simulink model "Practica5"  (R2020b)
settings: Solver=VariableStepAuto  StartTime=0.0  StopTime=10.0  RelTol=1e-3
values from neighbouring files (symbols this model uses):
  Cf = 0.0024    [Practica5Script.m]
  Fr = [10;0]    [Practica5Script.m]
  I = 0.0016    [Practica5Script.m]
  Ka = Ka(1)    [Practica5Script.m]
  Kd = [500 0;0 500]    [Practica5Script.m]
  Kp = Kp(1)    [Practica5Script.m]
  P = 0.00064    [Practica5Script.m]
undefined symbols (not defined in the file or in its folder): K, xe
settings Model: Creator=Danie  LastModifiedBy=Danie

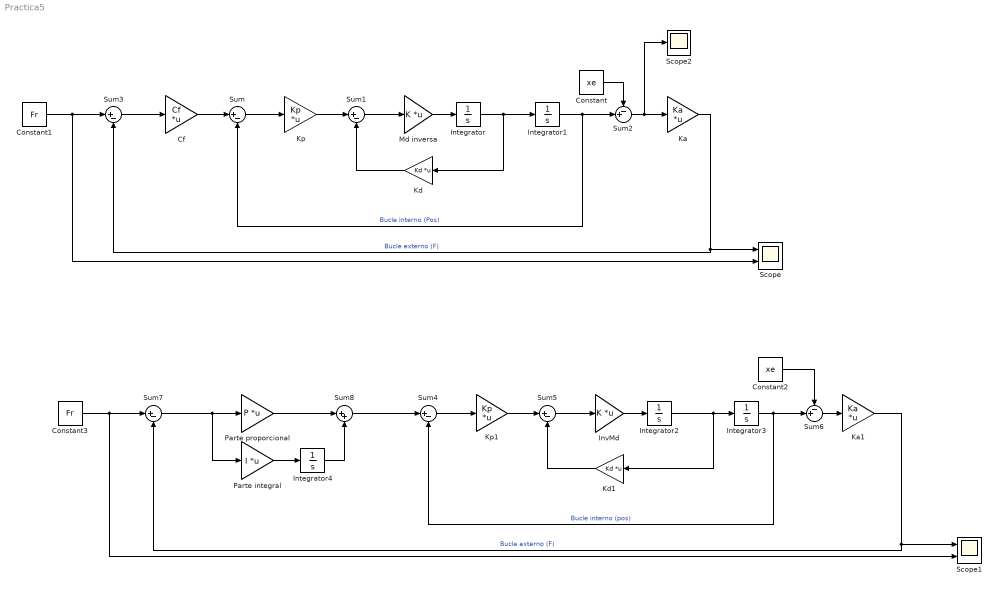
== system Practica5 ==
  Cf : Gain  Gain=Cf  Multiplication=Matrix(K*u)
  Constant : Constant  Value=xe
  Constant1 : Constant  Value=Fr
  Constant2 : Constant  Value=xe
  Constant3 : Constant  Value=Fr
  Integrator{,1..4} (5 alike) : Integrator
  InvMd : Gain  Gain=K  Multiplication=Matrix(K*u)
  Ka : Gain  Gain=Ka  Multiplication=Matrix(K*u)
  Ka1 : Gain  Gain=Ka  Multiplication=Matrix(K*u)
  Kd : Gain  Gain=Kd  Multiplication=Matrix(K*u)
  Kd1 : Gain  Gain=Kd  Multiplication=Matrix(K*u)
  Kp : Gain  Gain=Kp  Multiplication=Matrix(K*u)
  Kp1 : Gain  Gain=Kp  Multiplication=Matrix(K*u)
  Md inversa : Gain  Gain=K  Multiplication=Matrix(K*u)
  Parte integral : Gain  Gain=I  Multiplication=Matrix(K*u)
  "Parte proporcional " : Gain  Gain=P  Multiplication=Matrix(K*u)
  Scope : Scope  NumInputPorts=2
  Scope1 : Scope  NumInputPorts=2
  Scope2 : Scope
  Sum{,1,3..5,7} (6 alike) : Sum  Inputs=|+-
  Sum2 : Sum  Inputs=-+|
  Sum6 : Sum  Inputs=-+|
  Sum8 : Sum  Inputs=|++
  wires:
  Sum3/1 -> Cf/1
  Sum2/1 -> Scope2/1, Ka/1
  Md inversa/1 -> Integrator/1
  Sum/1 -> Kp/1
  Constant3/1 -> Scope1/2, Sum7/1
  Sum6/1 -> Ka1/1
  Parte integral/1 -> Integrator4/1
  Sum8/1 -> Sum4/1
  Sum5/1 -> InvMd/1
  Constant1/1 -> Scope/2, Sum3/1
  InvMd/1 -> Integrator2/1
  Kd/1 -> Sum1/2
  Integrator3/1 -> Sum6/2, Sum4/2  "Bucle interno (pos)"
  "Parte proporcional "/1 -> Sum8/1
  Kp1/1 -> Sum5/1
  Integrator2/1 -> Integrator3/1, Kd1/1
  Constant2/1 -> Sum6/1
  Ka/1 -> Sum3/2, Scope/1  "Bucle externo (F)"
  Constant/1 -> Sum2/1
  Integrator1/1 -> Sum2/2, Sum/2  "Bucle interno (Pos)"
  Sum1/1 -> Md inversa/1
  Integrator4/1 -> Sum8/2
  Integrator/1 -> Integrator1/1, Kd/1
  Kp/1 -> Sum1/1
  Cf/1 -> Sum/1
  Sum4/1 -> Kp1/1
  Kd1/1 -> Sum5/2
  Sum7/1 -> Parte integral/1, "Parte proporcional "/1
  Ka1/1 -> Scope1/1, Sum7/2  "Bucle externo (F)"
